simulink model "quarter_suspension_with_tire"  (R2020b)
settings: Solver=VariableStepAuto  StartTime=0.0  StopTime=5  RelTol=1e-3
values from neighbouring files (symbols this model uses):
  B_f = 1189    [halfcarparameters.mat]
  K = lqr(A,B,Q_pd,rho_pd)    [accel_jerk_ctrl_testbed.m]    (also in quartersuspensionscript.m)
  K_f = 66793    [halfcarparameters.mat]
  K_tf = 201021    [halfcarparameters.mat]
  m_s = 879.35    [halfcarparameters.mat]
  m_uf = 43.76    [halfcarparameters.mat]
settings Model: Creator=anishabhangui  LastModifiedBy=anishabhangui

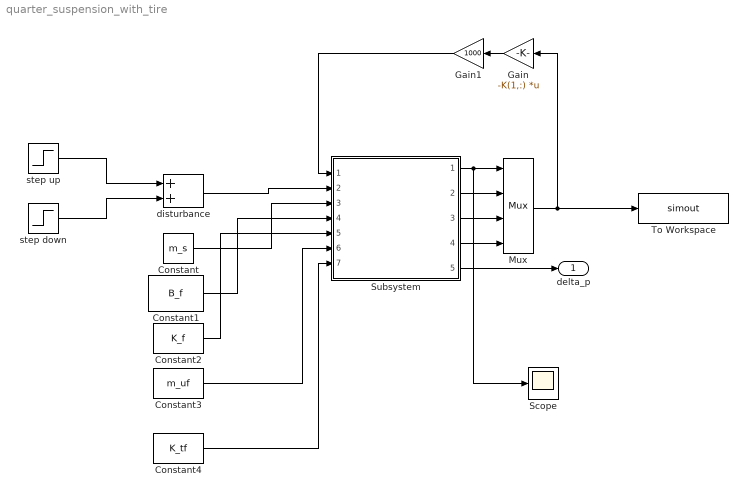
== system quarter_suspension_with_tire ==
  Constant : Constant  Value=m_s
  Constant1 : Constant  Value=B_f
  Constant2 : Constant  Value=K_f
  Constant3 : Constant  Value=m_uf
  Constant4 : Constant  Value=K_tf
  Gain : Gain  Gain=-K(1,:)  Multiplication=Matrix(K*u) (u vector)
  Gain1 : Gain  Gain=1000
  Mux : Mux
  Scope : Scope
  Subsystem : Subsystem  TreatAsAtomicUnit=on  ReferencedSubsystem=quarter_car_w_tire_subsystem
  To Workspace : ToWorkspace  VariableName=simout  SaveFormat=Timeseries  SampleTime=-1
  disturbance : Sum
  step down : Step  After=-1  SampleTime=0
  step up : Step  Time=0  SampleTime=0
  delta_p : Outport  VectorParamsAs1DForOutWhenUnconnected=off
  wires:
  Subsystem/5 -> delta_p/1
  step up/1 -> disturbance/1
  disturbance/1 -> Subsystem/2
  step down/1 -> disturbance/2
  Constant/1 -> Subsystem/3
  Constant1/1 -> Subsystem/4
  Constant2/1 -> Subsystem/5
  Constant3/1 -> Subsystem/6
  Constant4/1 -> Subsystem/7
  Subsystem/1 -> Scope/1, Mux/1
  Subsystem/2 -> Mux/2
  Subsystem/3 -> Mux/3
  Subsystem/4 -> Mux/4
  Mux/1 -> To Workspace/1, Gain/1
  Gain/1 -> Gain1/1
  Gain1/1 -> Subsystem/1
